simulink model "DHM"  (R2022a)
settings: Solver=FixedStepDiscrete  StartTime=0.0  StopTime=10.0  FixedStep=0.01  RelTol=1e-3
settings Model: Creator=DELL  LastModifiedBy=DELL
settings DataIOCC: SaveFormat=StructureWithTime
settings OptimizationCC: DefaultParameterBehavior=Inlined  EnhancedBackFolding=on  PassReuseOutputArgsAs=Individual arguments  ZeroExternalMemoryAtStartup=off  ZeroInternalMemoryAtStartup=off  OptimizeBlockOrder=speed  DifferentSizesBufferReuse=on  OptimizationCustomize=off  EfficientTunableParamExpr=on
settings DebuggingCC: ParameterTunabilityLossMsg=error
settings ModelReferenceCC: ModelReferenceNumInstancesAllowed=Single
settings SFSimCC: MATLABDynamicMemAlloc=off
settings RTWCC: Description=AUTOSAR  SystemTargetFile=autosar.tlc  GenCodeOnly=on  TemplateMakefile=ert_default_tmf
settings CodeAppCC: ForceParamTrailComments=on  IgnoreCustomStorageClasses=off  OperatorAnnotations=on  SimulinkDataObjDesc=on  SFDataObjDesc=on  InsertBlockDesc=on
settings STFCustomTargetCC: TargetLangStandard=C99 (ISO)  MultiwordLength=256  ParMdlRefBuildCompliant=on  CompOptLevelCompliant=on  IncludeMdlTerminateFcn=off  CombineOutputUpdateFcns=on  SuppressErrorStatus=on  ERTCustomFileBanners=on  SupportNonFinite=off  SupportComplex=off  SupportContinuousTime=off  SupportNonInlinedSFcns=off  RemoveResetFunc=on  MATLABClassNameForMDSCustomization=Simulink.SoftwareTarget.ERTCustomization  AutosarCompliant=on  GRTInterface=off  UseToolchainInfoCompliant=on  LookupTableObjectStructAxisOrder=2,1,3,4,...  LUTObjectStructOrderEvenSpacing=Size,Table,Breakpoints  SystemTargetFile=autosar.tlc
settings ERTTargetCC: TargetLangStandard=C99 (ISO)  ConcurrentExecutionCompliant=off  IncludeMdlTerminateFcn=off  SuppressErrorStatus=on  SupportNonFinite=off  SupportComplex=off  ModelStepFunctionPrototypeControlCompliant=off  CPPClassGenCompliant=off  AutosarCompliant=on  LookupTableObjectStructAxisOrder=2,1,3,4,...  LUTObjectStructOrderEvenSpacing=Size,Table,Breakpoints  InlinedParameterPlacement=NonHierarchical  ERTCustomFileTemplate=example_file_process.tlc

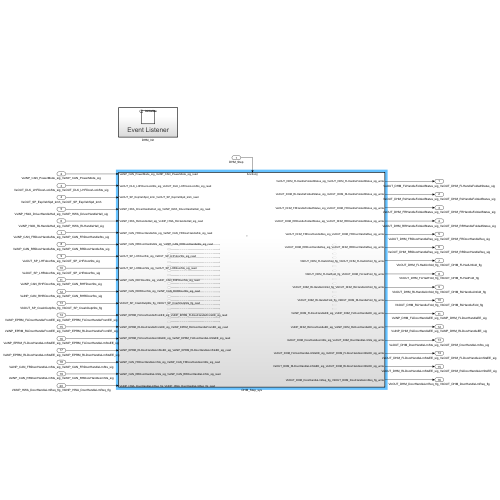
[thumbnail: Simulink's stored preview of the top-level diagram]
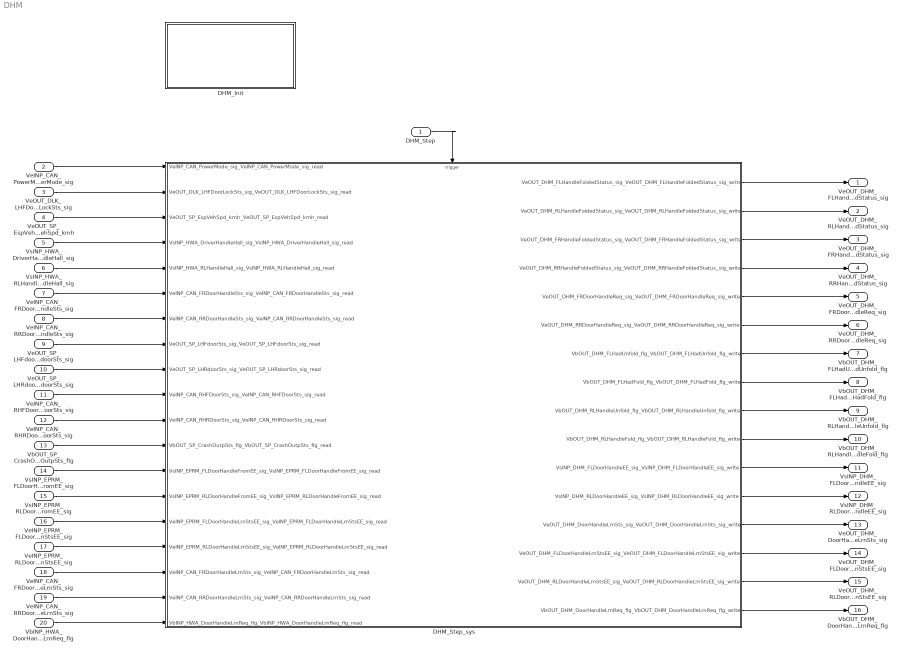
== system DHM ==
  DHM_Step : Inport  SampleTime=0.01  OutputFunctionCall=on
  VeINP_CAN_PowerMode_sig_VeINP_CAN_PowerMode_sig : Inport  Port=2  OutDataTypeStr=UInt8  PortDimensions=1
  VeOUT_DLK_LHFDoorLockSts_sig_VeOUT_DLK_LHFDoorLockSts_sig : Inport  Port=3  OutDataTypeStr=UInt8  PortDimensions=1
  VeOUT_SP_EspVehSpd_kmh_VeOUT_SP_EspVehSpd_kmh : Inport  Port=4  OutDataTypeStr=UInt8  PortDimensions=1
  VsINP_HWA_DriverHandleHall_sig_VsINP_HWA_DriverHandleHall_sig : Inport  Port=5  OutDataTypeStr=SInt16  PortDimensions=1
  VsINP_HWA_RLHandleHall_sig_VsINP_HWA_RLHandleHall_sig : Inport  Port=6  OutDataTypeStr=SInt16  PortDimensions=1
  VeINP_CAN_FRDoorHandleSts_sig_VeINP_CAN_FRDoorHandleSts_sig : Inport  Port=7  OutDataTypeStr=UInt8  PortDimensions=1
  VeINP_CAN_RRDoorHandleSts_sig_VeINP_CAN_RRDoorHandleSts_sig : Inport  Port=8  OutDataTypeStr=UInt8  PortDimensions=1
  VeOUT_SP_LHFdoorSts_sig_VeOUT_SP_LHFdoorSts_sig : Inport  Port=9  OutDataTypeStr=UInt8  PortDimensions=1
  VeOUT_SP_LHRdoorSts_sig_VeOUT_SP_LHRdoorSts_sig : Inport  Port=10  OutDataTypeStr=UInt8  PortDimensions=1
  VeINP_CAN_RHFDoorSts_sig_VeINP_CAN_RHFDoorSts_sig : Inport  Port=11  OutDataTypeStr=UInt8  PortDimensions=1
  VeINP_CAN_RHRDoorSts_sig_VeINP_CAN_RHRDoorSts_sig : Inport  Port=12  OutDataTypeStr=UInt8  PortDimensions=1
  VbOUT_SP_CrashOutpSts_flg_VbOUT_SP_CrashOutpSts_flg : Inport  Port=13  OutDataTypeStr=Boolean  PortDimensions=1
  VsINP_EPRM_FLDoorHandleFromEE_sig_VsINP_EPRM_FLDoorHandleFromEE_sig : Inport  Port=14  OutDataTypeStr=SInt16  PortDimensions=1
  VsINP_EPRM_RLDoorHandleFromEE_sig_VsINP_EPRM_RLDoorHandleFromEE_sig : Inport  Port=15  OutDataTypeStr=SInt16  PortDimensions=1
  VeINP_EPRM_FLDoorHandleLrnStsEE_sig_VeINP_EPRM_FLDoorHandleLrnStsEE_sig : Inport  Port=16  OutDataTypeStr=UInt8  PortDimensions=1
  VeINP_EPRM_RLDoorHandleLrnStsEE_sig_VeINP_EPRM_RLDoorHandleLrnStsEE_sig : Inport  Port=17  OutDataTypeStr=UInt8  PortDimensions=1
  VeINP_CAN_FRDoorHandleLrnSts_sig_VeINP_CAN_FRDoorHandleLrnSts_sig : Inport  Port=18  OutDataTypeStr=UInt8  PortDimensions=1
  VeINP_CAN_RRDoorHandleLrnSts_sig_VeINP_CAN_RRDoorHandleLrnSts_sig : Inport  Port=19  OutDataTypeStr=UInt8  PortDimensions=1
  VbINP_HWA_DoorHandleLrnReq_flg_VbINP_HWA_DoorHandleLrnReq_flg : Inport  Port=20  OutDataTypeStr=Boolean  PortDimensions=1
  DHM_Init : Subsystem
  DHM_Step_sys : Subsystem
  VeOUT_DHM_FLHandleFoldedStatus_sig_VeOUT_DHM_FLHandleFoldedStatus_sig : Outport  OutDataTypeStr=UInt8  PortDimensions=1
  VeOUT_DHM_RLHandleFoldedStatus_sig_VeOUT_DHM_RLHandleFoldedStatus_sig : Outport  Port=2  OutDataTypeStr=UInt8  PortDimensions=1
  VeOUT_DHM_FRHandleFoldedStatus_sig_VeOUT_DHM_FRHandleFoldedStatus_sig : Outport  Port=3  OutDataTypeStr=UInt8  PortDimensions=1
  VeOUT_DHM_RRHandleFoldedStatus_sig_VeOUT_DHM_RRHandleFoldedStatus_sig : Outport  Port=4  OutDataTypeStr=UInt8  PortDimensions=1
  VeOUT_DHM_FRDoorHandleReq_sig_VeOUT_DHM_FRDoorHandleReq_sig : Outport  Port=5  OutDataTypeStr=UInt8  PortDimensions=1
  VeOUT_DHM_RRDoorHandleReq_sig_VeOUT_DHM_RRDoorHandleReq_sig : Outport  Port=6  OutDataTypeStr=UInt8  PortDimensions=1
  VbOUT_DHM_FLHadUnfold_flg_VbOUT_DHM_FLHadUnfold_flg : Outport  Port=7  OutDataTypeStr=Boolean  PortDimensions=1
  VbOUT_DHM_FLHadFold_flg_VbOUT_DHM_FLHadFold_flg : Outport  Port=8  OutDataTypeStr=Boolean  PortDimensions=1
  VbOUT_DHM_RLHandleUnfold_flg_VbOUT_DHM_RLHandleUnfold_flg : Outport  Port=9  OutDataTypeStr=Boolean  PortDimensions=1
  VbOUT_DHM_RLHandleFold_flg_VbOUT_DHM_RLHandleFold_flg : Outport  Port=10  OutDataTypeStr=Boolean  PortDimensions=1
  VsINP_DHM_FLDoorHandleEE_sig_VsINP_DHM_FLDoorHandleEE_sig : Outport  Port=11  OutDataTypeStr=SInt16  PortDimensions=1
  VsINP_DHM_RLDoorHandleEE_sig_VsINP_DHM_RLDoorHandleEE_sig : Outport  Port=12  OutDataTypeStr=SInt16  PortDimensions=1
  VeOUT_DHM_DoorHandleLrnSts_sig_VeOUT_DHM_DoorHandleLrnSts_sig : Outport  Port=13  OutDataTypeStr=UInt8  PortDimensions=1
  VeOUT_DHM_FLDoorHandleLrnStsEE_sig_VeOUT_DHM_FLDoorHandleLrnStsEE_sig : Outport  Port=14  OutDataTypeStr=UInt8  PortDimensions=1
  VeOUT_DHM_RLDoorHandleLrnStsEE_sig_VeOUT_DHM_RLDoorHandleLrnStsEE_sig : Outport  Port=15  OutDataTypeStr=UInt8  PortDimensions=1
  VbOUT_DHM_DoorHandleLrnReq_flg_VbOUT_DHM_DoorHandleLrnReq_flg : Outport  Port=16  OutDataTypeStr=Boolean  PortDimensions=1
  wires:
  VeINP_CAN_PowerMode_sig_VeINP_CAN_PowerMode_sig/1 -> DHM_Step_sys/1(VeINP_CAN_PowerMode_sig_VeINP_CAN_PowerMode_sig_read)
  VeOUT_DLK_LHFDoorLockSts_sig_VeOUT_DLK_LHFDoorLockSts_sig/1 -> DHM_Step_sys/2(VeOUT_DLK_LHFDoorLockSts_sig_VeOUT_DLK_LHFDoorLockSts_sig_read)
  VeOUT_SP_EspVehSpd_kmh_VeOUT_SP_EspVehSpd_kmh/1 -> DHM_Step_sys/3(VeOUT_SP_EspVehSpd_kmh_VeOUT_SP_EspVehSpd_kmh_read)
  VsINP_HWA_DriverHandleHall_sig_VsINP_HWA_DriverHandleHall_sig/1 -> DHM_Step_sys/4(VsINP_HWA_DriverHandleHall_sig_VsINP_HWA_DriverHandleHall_sig_read)
  VsINP_HWA_RLHandleHall_sig_VsINP_HWA_RLHandleHall_sig/1 -> DHM_Step_sys/5(VsINP_HWA_RLHandleHall_sig_VsINP_HWA_RLHandleHall_sig_read)
  VeINP_CAN_FRDoorHandleSts_sig_VeINP_CAN_FRDoorHandleSts_sig/1 -> DHM_Step_sys/6(VeINP_CAN_FRDoorHandleSts_sig_VeINP_CAN_FRDoorHandleSts_sig_read)
  VeINP_CAN_RRDoorHandleSts_sig_VeINP_CAN_RRDoorHandleSts_sig/1 -> DHM_Step_sys/7(VeINP_CAN_RRDoorHandleSts_sig_VeINP_CAN_RRDoorHandleSts_sig_read)
  VeOUT_SP_LHFdoorSts_sig_VeOUT_SP_LHFdoorSts_sig/1 -> DHM_Step_sys/8(VeOUT_SP_LHFdoorSts_sig_VeOUT_SP_LHFdoorSts_sig_read)
  VeOUT_SP_LHRdoorSts_sig_VeOUT_SP_LHRdoorSts_sig/1 -> DHM_Step_sys/9(VeOUT_SP_LHRdoorSts_sig_VeOUT_SP_LHRdoorSts_sig_read)
  VeINP_CAN_RHFDoorSts_sig_VeINP_CAN_RHFDoorSts_sig/1 -> DHM_Step_sys/10(VeINP_CAN_RHFDoorSts_sig_VeINP_CAN_RHFDoorSts_sig_read)
  VeINP_CAN_RHRDoorSts_sig_VeINP_CAN_RHRDoorSts_sig/1 -> DHM_Step_sys/11(VeINP_CAN_RHRDoorSts_sig_VeINP_CAN_RHRDoorSts_sig_read)
  VbOUT_SP_CrashOutpSts_flg_VbOUT_SP_CrashOutpSts_flg/1 -> DHM_Step_sys/12(VbOUT_SP_CrashOutpSts_flg_VbOUT_SP_CrashOutpSts_flg_read)
  VsINP_EPRM_FLDoorHandleFromEE_sig_VsINP_EPRM_FLDoorHandleFromEE_sig/1 -> DHM_Step_sys/13(VsINP_EPRM_FLDoorHandleFromEE_sig_VsINP_EPRM_FLDoorHandleFromEE_sig_read)
  VsINP_EPRM_RLDoorHandleFromEE_sig_VsINP_EPRM_RLDoorHandleFromEE_sig/1 -> DHM_Step_sys/14(VsINP_EPRM_RLDoorHandleFromEE_sig_VsINP_EPRM_RLDoorHandleFromEE_sig_read)
  VeINP_EPRM_FLDoorHandleLrnStsEE_sig_VeINP_EPRM_FLDoorHandleLrnStsEE_sig/1 -> DHM_Step_sys/15(VeINP_EPRM_FLDoorHandleLrnStsEE_sig_VeINP_EPRM_FLDoorHandleLrnStsEE_sig_read)
  VeINP_EPRM_RLDoorHandleLrnStsEE_sig_VeINP_EPRM_RLDoorHandleLrnStsEE_sig/1 -> DHM_Step_sys/16(VeINP_EPRM_RLDoorHandleLrnStsEE_sig_VeINP_EPRM_RLDoorHandleLrnStsEE_sig_read)
  VeINP_CAN_FRDoorHandleLrnSts_sig_VeINP_CAN_FRDoorHandleLrnSts_sig/1 -> DHM_Step_sys/17(VeINP_CAN_FRDoorHandleLrnSts_sig_VeINP_CAN_FRDoorHandleLrnSts_sig_read)
  VeINP_CAN_RRDoorHandleLrnSts_sig_VeINP_CAN_RRDoorHandleLrnSts_sig/1 -> DHM_Step_sys/18(VeINP_CAN_RRDoorHandleLrnSts_sig_VeINP_CAN_RRDoorHandleLrnSts_sig_read)
  VbINP_HWA_DoorHandleLrnReq_flg_VbINP_HWA_DoorHandleLrnReq_flg/1 -> DHM_Step_sys/19(VbINP_HWA_DoorHandleLrnReq_flg_VbINP_HWA_DoorHandleLrnReq_flg_read)
  DHM_Step_sys/1(VeOUT_DHM_FLHandleFoldedStatus_sig_VeOUT_DHM_FLHandleFoldedStatus_sig_write) -> VeOUT_DHM_FLHandleFoldedStatus_sig_VeOUT_DHM_FLHandleFoldedStatus_sig/1
  DHM_Step_sys/2(VeOUT_DHM_RLHandleFoldedStatus_sig_VeOUT_DHM_RLHandleFoldedStatus_sig_write) -> VeOUT_DHM_RLHandleFoldedStatus_sig_VeOUT_DHM_RLHandleFoldedStatus_sig/1
  DHM_Step_sys/3(VeOUT_DHM_FRHandleFoldedStatus_sig_VeOUT_DHM_FRHandleFoldedStatus_sig_write) -> VeOUT_DHM_FRHandleFoldedStatus_sig_VeOUT_DHM_FRHandleFoldedStatus_sig/1
  DHM_Step_sys/4(VeOUT_DHM_RRHandleFoldedStatus_sig_VeOUT_DHM_RRHandleFoldedStatus_sig_write) -> VeOUT_DHM_RRHandleFoldedStatus_sig_VeOUT_DHM_RRHandleFoldedStatus_sig/1
  DHM_Step_sys/5(VeOUT_DHM_FRDoorHandleReq_sig_VeOUT_DHM_FRDoorHandleReq_sig_write) -> VeOUT_DHM_FRDoorHandleReq_sig_VeOUT_DHM_FRDoorHandleReq_sig/1
  DHM_Step_sys/6(VeOUT_DHM_RRDoorHandleReq_sig_VeOUT_DHM_RRDoorHandleReq_sig_write) -> VeOUT_DHM_RRDoorHandleReq_sig_VeOUT_DHM_RRDoorHandleReq_sig/1
  DHM_Step_sys/7(VbOUT_DHM_FLHadUnfold_flg_VbOUT_DHM_FLHadUnfold_flg_write) -> VbOUT_DHM_FLHadUnfold_flg_VbOUT_DHM_FLHadUnfold_flg/1
  DHM_Step_sys/8(VbOUT_DHM_FLHadFold_flg_VbOUT_DHM_FLHadFold_flg_write) -> VbOUT_DHM_FLHadFold_flg_VbOUT_DHM_FLHadFold_flg/1
  DHM_Step_sys/9(VbOUT_DHM_RLHandleUnfold_flg_VbOUT_DHM_RLHandleUnfold_flg_write) -> VbOUT_DHM_RLHandleUnfold_flg_VbOUT_DHM_RLHandleUnfold_flg/1
  DHM_Step_sys/10(VbOUT_DHM_RLHandleFold_flg_VbOUT_DHM_RLHandleFold_flg_write) -> VbOUT_DHM_RLHandleFold_flg_VbOUT_DHM_RLHandleFold_flg/1
  DHM_Step_sys/11(VsINP_DHM_FLDoorHandleEE_sig_VsINP_DHM_FLDoorHandleEE_sig_write) -> VsINP_DHM_FLDoorHandleEE_sig_VsINP_DHM_FLDoorHandleEE_sig/1
  DHM_Step_sys/12(VsINP_DHM_RLDoorHandleEE_sig_VsINP_DHM_RLDoorHandleEE_sig_write) -> VsINP_DHM_RLDoorHandleEE_sig_VsINP_DHM_RLDoorHandleEE_sig/1
  DHM_Step_sys/13(VeOUT_DHM_DoorHandleLrnSts_sig_VeOUT_DHM_DoorHandleLrnSts_sig_write) -> VeOUT_DHM_DoorHandleLrnSts_sig_VeOUT_DHM_DoorHandleLrnSts_sig/1
  DHM_Step_sys/14(VeOUT_DHM_FLDoorHandleLrnStsEE_sig_VeOUT_DHM_FLDoorHandleLrnStsEE_sig_write) -> VeOUT_DHM_FLDoorHandleLrnStsEE_sig_VeOUT_DHM_FLDoorHandleLrnStsEE_sig/1
  DHM_Step_sys/15(VeOUT_DHM_RLDoorHandleLrnStsEE_sig_VeOUT_DHM_RLDoorHandleLrnStsEE_sig_write) -> VeOUT_DHM_RLDoorHandleLrnStsEE_sig_VeOUT_DHM_RLDoorHandleLrnStsEE_sig/1
  DHM_Step_sys/16(VbOUT_DHM_DoorHandleLrnReq_flg_VbOUT_DHM_DoorHandleLrnReq_flg_write) -> VbOUT_DHM_DoorHandleLrnReq_flg_VbOUT_DHM_DoorHandleLrnReq_flg/1
  DHM_Step/1 -> DHM_Step_sys/Trigger

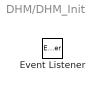
== system DHM/DHM_Init ==
  Event Listener : EventListener  EventName=reset

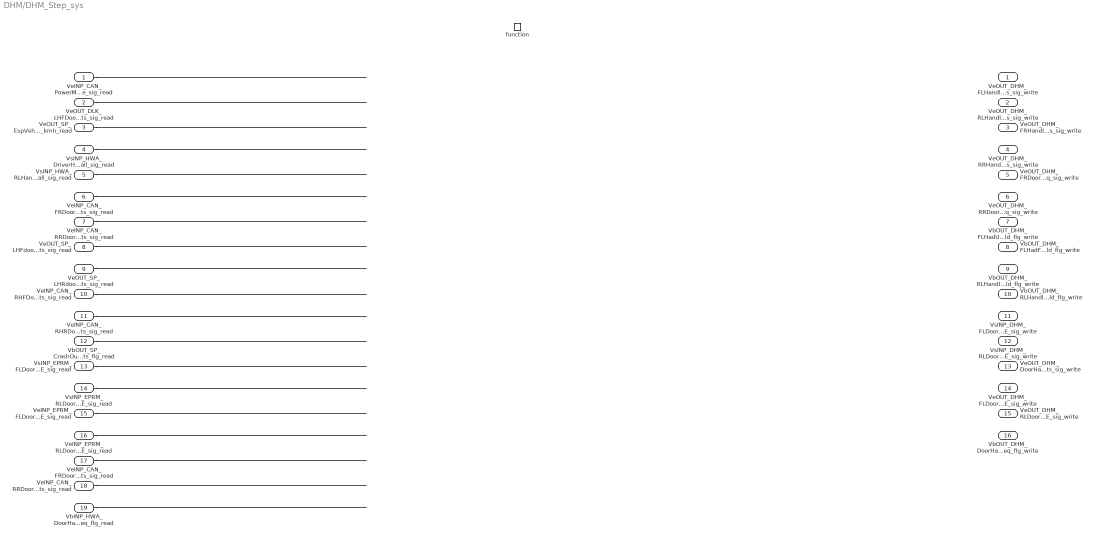
== system DHM/DHM_Step_sys ==
  VeINP_CAN_PowerMode_sig_VeINP_CAN_PowerMode_sig_read : Inport
  VeOUT_DLK_LHFDoorLockSts_sig_VeOUT_DLK_LHFDoorLockSts_sig_read : Inport  Port=2
  VeOUT_SP_EspVehSpd_kmh_VeOUT_SP_EspVehSpd_kmh_read : Inport  Port=3
  VsINP_HWA_DriverHandleHall_sig_VsINP_HWA_DriverHandleHall_sig_read : Inport  Port=4
  VsINP_HWA_RLHandleHall_sig_VsINP_HWA_RLHandleHall_sig_read : Inport  Port=5
  VeINP_CAN_FRDoorHandleSts_sig_VeINP_CAN_FRDoorHandleSts_sig_read : Inport  Port=6
  VeINP_CAN_RRDoorHandleSts_sig_VeINP_CAN_RRDoorHandleSts_sig_read : Inport  Port=7
  VeOUT_SP_LHFdoorSts_sig_VeOUT_SP_LHFdoorSts_sig_read : Inport  Port=8
  VeOUT_SP_LHRdoorSts_sig_VeOUT_SP_LHRdoorSts_sig_read : Inport  Port=9
  VeINP_CAN_RHFDoorSts_sig_VeINP_CAN_RHFDoorSts_sig_read : Inport  Port=10
  VeINP_CAN_RHRDoorSts_sig_VeINP_CAN_RHRDoorSts_sig_read : Inport  Port=11
  VbOUT_SP_CrashOutpSts_flg_VbOUT_SP_CrashOutpSts_flg_read : Inport  Port=12
  VsINP_EPRM_FLDoorHandleFromEE_sig_VsINP_EPRM_FLDoorHandleFromEE_sig_read : Inport  Port=13
  VsINP_EPRM_RLDoorHandleFromEE_sig_VsINP_EPRM_RLDoorHandleFromEE_sig_read : Inport  Port=14
  VeINP_EPRM_FLDoorHandleLrnStsEE_sig_VeINP_EPRM_FLDoorHandleLrnStsEE_sig_read : Inport  Port=15
  VeINP_EPRM_RLDoorHandleLrnStsEE_sig_VeINP_EPRM_RLDoorHandleLrnStsEE_sig_read : Inport  Port=16
  VeINP_CAN_FRDoorHandleLrnSts_sig_VeINP_CAN_FRDoorHandleLrnSts_sig_read : Inport  Port=17
  VeINP_CAN_RRDoorHandleLrnSts_sig_VeINP_CAN_RRDoorHandleLrnSts_sig_read : Inport  Port=18
  VbINP_HWA_DoorHandleLrnReq_flg_VbINP_HWA_DoorHandleLrnReq_flg_read : Inport  Port=19
  function : TriggerPort  TriggerType=function-call  VariantControl=(inherit)  SampleTimeType=periodic  SampleTime=-1
  VeOUT_DHM_FLHandleFoldedStatus_sig_VeOUT_DHM_FLHandleFoldedStatus_sig_write : Outport
      settings: EnsureOutportIsVirtual=on
  VeOUT_DHM_RLHandleFoldedStatus_sig_VeOUT_DHM_RLHandleFoldedStatus_sig_write : Outport  Port=2
      settings: EnsureOutportIsVirtual=on
  VeOUT_DHM_FRHandleFoldedStatus_sig_VeOUT_DHM_FRHandleFoldedStatus_sig_write : Outport  Port=3
      settings: EnsureOutportIsVirtual=on
  VeOUT_DHM_RRHandleFoldedStatus_sig_VeOUT_DHM_RRHandleFoldedStatus_sig_write : Outport  Port=4
      settings: EnsureOutportIsVirtual=on
  VeOUT_DHM_FRDoorHandleReq_sig_VeOUT_DHM_FRDoorHandleReq_sig_write : Outport  Port=5
      settings: EnsureOutportIsVirtual=on
  VeOUT_DHM_RRDoorHandleReq_sig_VeOUT_DHM_RRDoorHandleReq_sig_write : Outport  Port=6
      settings: EnsureOutportIsVirtual=on
  VbOUT_DHM_FLHadUnfold_flg_VbOUT_DHM_FLHadUnfold_flg_write : Outport  Port=7
      settings: EnsureOutportIsVirtual=on
  VbOUT_DHM_FLHadFold_flg_VbOUT_DHM_FLHadFold_flg_write : Outport  Port=8
      settings: EnsureOutportIsVirtual=on
  VbOUT_DHM_RLHandleUnfold_flg_VbOUT_DHM_RLHandleUnfold_flg_write : Outport  Port=9
      settings: EnsureOutportIsVirtual=on
  VbOUT_DHM_RLHandleFold_flg_VbOUT_DHM_RLHandleFold_flg_write : Outport  Port=10
      settings: EnsureOutportIsVirtual=on
  VsINP_DHM_FLDoorHandleEE_sig_VsINP_DHM_FLDoorHandleEE_sig_write : Outport  Port=11
      settings: EnsureOutportIsVirtual=on
  VsINP_DHM_RLDoorHandleEE_sig_VsINP_DHM_RLDoorHandleEE_sig_write : Outport  Port=12
      settings: EnsureOutportIsVirtual=on
  VeOUT_DHM_DoorHandleLrnSts_sig_VeOUT_DHM_DoorHandleLrnSts_sig_write : Outport  Port=13
      settings: EnsureOutportIsVirtual=on
  VeOUT_DHM_FLDoorHandleLrnStsEE_sig_VeOUT_DHM_FLDoorHandleLrnStsEE_sig_write : Outport  Port=14
      settings: EnsureOutportIsVirtual=on
  VeOUT_DHM_RLDoorHandleLrnStsEE_sig_VeOUT_DHM_RLDoorHandleLrnStsEE_sig_write : Outport  Port=15
      settings: EnsureOutportIsVirtual=on
  VbOUT_DHM_DoorHandleLrnReq_flg_VbOUT_DHM_DoorHandleLrnReq_flg_write : Outport  Port=16
      settings: EnsureOutportIsVirtual=on
  wires:
  VeINP_CAN_PowerMode_sig_VeINP_CAN_PowerMode_sig_read/1 -> ?
  VeOUT_DLK_LHFDoorLockSts_sig_VeOUT_DLK_LHFDoorLockSts_sig_read/1 -> ?
  VeOUT_SP_EspVehSpd_kmh_VeOUT_SP_EspVehSpd_kmh_read/1 -> ?
  VsINP_HWA_DriverHandleHall_sig_VsINP_HWA_DriverHandleHall_sig_read/1 -> ?
  VsINP_HWA_RLHandleHall_sig_VsINP_HWA_RLHandleHall_sig_read/1 -> ?
  VeINP_CAN_FRDoorHandleSts_sig_VeINP_CAN_FRDoorHandleSts_sig_read/1 -> ?
  VeINP_CAN_RRDoorHandleSts_sig_VeINP_CAN_RRDoorHandleSts_sig_read/1 -> ?
  VeOUT_SP_LHFdoorSts_sig_VeOUT_SP_LHFdoorSts_sig_read/1 -> ?
  VeOUT_SP_LHRdoorSts_sig_VeOUT_SP_LHRdoorSts_sig_read/1 -> ?
  VeINP_CAN_RHFDoorSts_sig_VeINP_CAN_RHFDoorSts_sig_read/1 -> ?
  VeINP_CAN_RHRDoorSts_sig_VeINP_CAN_RHRDoorSts_sig_read/1 -> ?
  VbOUT_SP_CrashOutpSts_flg_VbOUT_SP_CrashOutpSts_flg_read/1 -> ?
  VsINP_EPRM_FLDoorHandleFromEE_sig_VsINP_EPRM_FLDoorHandleFromEE_sig_read/1 -> ?
  VsINP_EPRM_RLDoorHandleFromEE_sig_VsINP_EPRM_RLDoorHandleFromEE_sig_read/1 -> ?
  VeINP_EPRM_FLDoorHandleLrnStsEE_sig_VeINP_EPRM_FLDoorHandleLrnStsEE_sig_read/1 -> ?
  VeINP_EPRM_RLDoorHandleLrnStsEE_sig_VeINP_EPRM_RLDoorHandleLrnStsEE_sig_read/1 -> ?
  VeINP_CAN_FRDoorHandleLrnSts_sig_VeINP_CAN_FRDoorHandleLrnSts_sig_read/1 -> ?
  VeINP_CAN_RRDoorHandleLrnSts_sig_VeINP_CAN_RRDoorHandleLrnSts_sig_read/1 -> ?
  VbINP_HWA_DoorHandleLrnReq_flg_VbINP_HWA_DoorHandleLrnReq_flg_read/1 -> ?
